simulink model "FMC_TopLevel_Model_2025a"  (R2025a)
settings: Solver=ode23s  StartTime=0.0  StopTime=10.0  RelTol=1e-3
libraries: nesl_utility x1
settings Model: Creator=mu22504  LastModifiedBy=dj23106
settings DataIOCC: InspectSignalLogs=on
settings SimscapeCC: SimscapeLogType=all  SimscapeLogSimulationStatistics=on  SimscapeLogToSDI=on

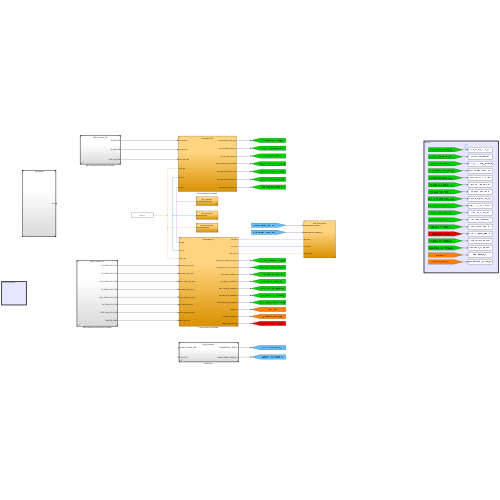
[thumbnail: Simulink's stored preview of the top-level diagram]
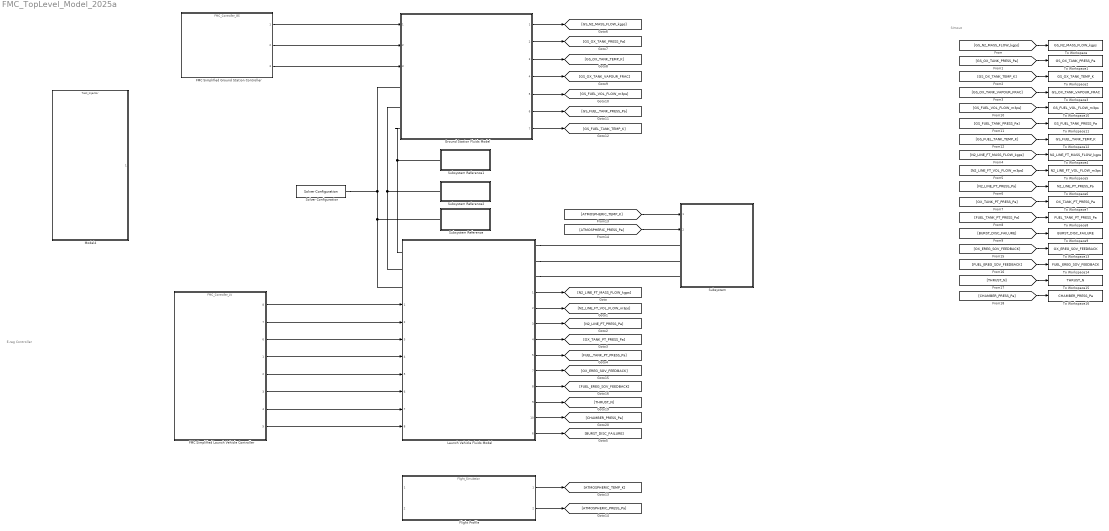
== system FMC_TopLevel_Model_2025a ==
  note: SImout
  note: E-reg Controller
  FMC Simplified Ground Station Controller : ModelReference  ModelNameDialog=FMC_Controller_GS  SimulationMode=Normal  ModelReferenceVersion=1.3
  FMC Simplified Launch Vehicle Controller : ModelReference  ModelNameDialog=FMC_Controller_LV  SimulationMode=Normal  ModelReferenceVersion=1.5
      settings: PortSchema="{\"entries\":[{\"content\":{\"sides\":[{\"content\":{},\"type\":\"ConnectorPlacement.EquallySpacedRectSide\",\"uuid\":\"d1f82117-a1a8-406f-b4c0-5c69a1a9a37f\"},{\"content\":{\"connectorIds\":[\"Out8\",\"Out7\",\"Out6\",\"Out1\",\"Out2\",\"Out3\",\"Out4\",\"Out5\"],\"side\":\"RIGHT\"},\"type\":\"ConnectorPlacement.EquallySpacedRectSide\",\"uuid\":\"19edbef6-afc0-4598-9a4a-36dbc083b03b\"},{\"content\":{\"side\":\"TOP\"},\"type\":\"ConnectorPlacement.EquallySpacedRectSide\",\"uuid\":\"6f6c62f6-4d0e-4b54-92d5-ff51912a203d\"}]},\"type\":\"ConnectorPlacement.EquallySpacedConnector\",\"uuid\":\"dc15e51f-b1bc-449a-a4f6-d80e0204dd3c\"}],\"packageUris\":[\"http://schema.mathworks.com/mf0/Connector/R2020b\"],\"version\":\"1.0\"}"
  "Flight Profile " : ModelReference  ModelNameDialog=Flight_Simulation.slx  SimulationMode=Normal  ModelReferenceVersion=1.3
  Ground Station Fluids Model : Subsystem  ReferencedSubsystem=Thermofluids_GS
      settings: PortSchema="{\"entries\":[{\"content\":{\"sides\":[{\"content\":{\"connectorIds\":[\"In1\",\"In2\",\"In3\",\"LConn3\",\"LConn2\",\"LConn1\"]},\"type\":\"ConnectorPlacement.EquallySpacedRectSide\",\"uuid\":\"1f0e9dc9-066f-4740-a01f-c871041edae1\"},{\"content\":{\"connectorIds\":[\"Out1\",\"Out2\",\"Out3\",\"Out4\",\"Out5\",\"Out6\",\"Out7\"],\"side\":\"RIGHT\"},\"type\":\"ConnectorPlacement.EquallySpacedRectSide\",\"uuid\":\"23696615-9e6b-4b01-bf34-3e6084e0acc4\"},{\"content\":{\"side\":\"TOP\"},\"type\":\"ConnectorPlacement.EquallySpacedRectSide\",\"uuid\":\"47968613-aa29-4234-9156-172438f99733\"}]},\"type\":\"ConnectorPlacement.EquallySpacedConnector\",\"uuid\":\"3d468e28-1aed-4784-9850-3053ce02f939\"}],\"packageUris\":[\"http://schema.mathworks.com/mf0/Connector/R2020b\"],\"version\":\"1.0\"}"
  Launch Vehicle Fluids Model : Subsystem  ReferencedSubsystem=Thermofluids_LV
      settings: PortSchema="{\"entries\":[{\"content\":{\"sides\":[{\"content\":{\"connectorIds\":[\"LConn1\",\"LConn2\",\"LConn3\",\"In1\",\"In2\",\"In3\",\"In4\",\"In5\",\"In6\",\"In7\",\"In8\"]},\"type\":\"ConnectorPlacement.EquallySpacedRectSide\",\"uuid\":\"a87b0425-c6b8-4d08-a1a8-b3acad5c334a\"},{\"content\":{\"connectorIds\":[\"LConn4\",\"LConn5\",\"LConn6\",\"Out1\",\"Out2\",\"Out3\",\"Out4\",\"Out5\",\"Out7\",\"Out8\",\"Out9\",\"Out10\",\"Out6\"],\"side\":\"RIGHT\"},\"type\":\"ConnectorPlacement.EquallySpacedRectSide\",\"uuid\":\"260d6155-6d20-4ed3-9052-698506ea1559\"},{\"content\":{\"side\":\"TOP\"},\"type\":\"ConnectorPlacement.EquallySpacedRectSide\",\"uuid\":\"d266d02d-922b-4f41-b529-513bc445e931\"}]},\"type\":\"ConnectorPlacement.EquallySpacedConnector\",\"uuid\":\"36f51c95-b9e3-4232-bda9-d5a6ea8a2ffc\"}],\"packageUris\":[\"http://schema.mathworks.com/mf0/Connector/R2020b\"],\"version\":\"1.0\"}"
  Model4 : ModelReference  ModelNameDialog=Test_Injector.slx  SimulationMode=Normal  ModelReferenceVersion=1.3
  Solver Configuration : nesl_utility/Solver Configuration  PhysicalDomain=network_engine_domain  SubClassName=solver  LeftPortType=input  RightPortType=generic  Tones=[]  Harmonics=[]  SimulateNoise=off  Profile=off  UseLocalSampling=off  EnableSwitchedLinearOptims=on  FrequencyDomain=off  UseCCode=off  RelTol=0.001  AbsTol=0.001  MinStep=1e-09  ToWorkspace=off  RevertToSquareIcSolve=off  NumHomotopyIterations=100  PhasorMode=off  PhasorModeNumHarmonics=1  ConsistencySolver=NEWTON_XTOL_AFTER_FTOL  IndexReductionMethod=DerivativeReplacement  DoDC=off  ResidualTolerance=1e-09  ConsistencyTolSource=GLOBAL  ConsistencyAbsTol=0.001  ConsistencyRelTol=0.001  ConsistencyTolFactor=0.001  UseLocalSolver=off  LocalSolverChoice=NE_BACKWARD_EULER_ADVANCER  ResolveIndetEquations=on  FunctionEvalNumThread=1  LocalSolverSampleTime=0.001  DoFixedCost=off  MaxNonlinIter=3  MaxModeIter=2  ComputeImpulses=off  ImpulseIterations=2  LinearAlgebra=auto  LinearAlgebraNumThread=0  EquationFormulation=NE_TIME_EF  DelaysMemoryBudget=1024  AutomaticFiltering=on  FilteringTimeConstant=0.001  PartitionStorageMethod=AS_NEEDED  PartitionMemoryBudget=1024  PartitionMethod=ROBUST  MultibodyUseLocalSolver=off  MultibodyLocalSolverChoice=ODE1  MultibodyLocalSolverSampleTime=0.001
  Subsystem : Subsystem  ReferencedSubsystem=Vent_Environment
  Subsystem Reference : Subsystem  ReferencedSubsystem=ethanol_properties
  Subsystem Reference1 : Subsystem  ReferencedSubsystem=N2_properties
  Subsystem Reference2 : Subsystem  ReferencedSubsystem=N2O_properties
  To Workspace : ToWorkspace  VariableName=GS_N2_MASS_FLOW_kgps  SaveFormat=Timeseries  SampleTime=-1
  To Workspace1 : ToWorkspace  VariableName=GS_OX_TANK_PRESS_Pa  SaveFormat=Timeseries  SampleTime=-1
  To Workspace10 : ToWorkspace  VariableName=GS_FUEL_VOL_FLOW_m3ps  SaveFormat=Timeseries  SampleTime=-1
  To Workspace11 : ToWorkspace  VariableName=GS_FUEL_TANK_PRESS_Pa  SaveFormat=Timeseries  SampleTime=-1
  To Workspace12 : ToWorkspace  VariableName=GS_FUEL_TANK_TEMP_K  SaveFormat=Timeseries  SampleTime=-1
  To Workspace13 : ToWorkspace  VariableName=OX_EREG_SOV_FEEDBACK  SaveFormat=Timeseries  SampleTime=-1
  To Workspace14 : ToWorkspace  VariableName=FUEL_EREG_SOV_FEEDBACK  SaveFormat=Timeseries  SampleTime=-1
  To Workspace15 : ToWorkspace  VariableName=THRUST_N  SaveFormat=Timeseries  SampleTime=-1
  To Workspace16 : ToWorkspace  VariableName=CHAMBER_PRESS_Pa  SaveFormat=Timeseries  SampleTime=-1
  To Workspace2 : ToWorkspace  VariableName=GS_OX_TANK_TEMP_K  SaveFormat=Timeseries  SampleTime=-1
  To Workspace3 : ToWorkspace  VariableName=GS_OX_TANK_VAPOUR_FRAC  SaveFormat=Timeseries  SampleTime=-1
  To Workspace4 : ToWorkspace  VariableName=N2_LINE_FT_MASS_FLOW_kgps  SaveFormat=Timeseries  SampleTime=-1
  To Workspace5 : ToWorkspace  VariableName=N2_LINE_FT_VOL_FLOW_m3ps  SaveFormat=Timeseries  SampleTime=-1
  To Workspace6 : ToWorkspace  VariableName=N2_LINE_PT_PRESS_Pa  SaveFormat=Timeseries  SampleTime=-1
  To Workspace7 : ToWorkspace  VariableName=OX_TANK_PT_PRESS_Pa  SaveFormat=Timeseries  SampleTime=-1
  To Workspace8 : ToWorkspace  VariableName=FUEL_TANK_PT_PRESS_Pa  SaveFormat=Timeseries  SampleTime=-1
  To Workspace9 : ToWorkspace  VariableName=BURST_DISC_FAILURE  SaveFormat=Timeseries  SampleTime=-1
  wires:
  Launch Vehicle Fluids Model/1 -> [N2_LINE_FT_MASS_FLOW_kgps]
  Launch Vehicle Fluids Model/2 -> [N2_LINE_FT_VOL_FLOW_m3ps]
  Launch Vehicle Fluids Model/3 -> [N2_LINE_PT_PRESS_Pa]
  Launch Vehicle Fluids Model/4 -> [OX_TANK_PT_PRESS_Pa]
  Launch Vehicle Fluids Model/5 -> [FUEL_TANK_PT_PRESS_Pa]
  Launch Vehicle Fluids Model/6 -> [BURST_DISC_FAILURE]
  FMC Simplified Ground Station Controller/1 -> Ground Station Fluids Model/1
  FMC Simplified Ground Station Controller/2 -> Ground Station Fluids Model/2
  FMC Simplified Ground Station Controller/3 -> Ground Station Fluids Model/3
  Ground Station Fluids Model/1 -> [GS_N2_MASS_FLOW_kgps]
  Ground Station Fluids Model/2 -> [GS_OX_TANK_PRESS_Pa]
  Ground Station Fluids Model/3 -> [GS_OX_TANK_TEMP_K]
  Ground Station Fluids Model/4 -> [GS_OX_TANK_VAPOUR_FRAC]
  [GS_N2_MASS_FLOW_kgps] -> To Workspace/1
  [GS_OX_TANK_PRESS_Pa] -> To Workspace1/1
  [GS_OX_TANK_TEMP_K] -> To Workspace2/1
  [GS_OX_TANK_VAPOUR_FRAC] -> To Workspace3/1
  [N2_LINE_FT_MASS_FLOW_kgps] -> To Workspace4/1
  [BURST_DISC_FAILURE] -> To Workspace9/1
  [FUEL_TANK_PT_PRESS_Pa] -> To Workspace8/1
  [OX_TANK_PT_PRESS_Pa] -> To Workspace7/1
  [N2_LINE_PT_PRESS_Pa] -> To Workspace6/1
  [N2_LINE_FT_VOL_FLOW_m3ps] -> To Workspace5/1
  FMC Simplified Launch Vehicle Controller/5 -> Launch Vehicle Fluids Model/8
  FMC Simplified Launch Vehicle Controller/4 -> Launch Vehicle Fluids Model/7
  FMC Simplified Launch Vehicle Controller/3 -> Launch Vehicle Fluids Model/6
  FMC Simplified Launch Vehicle Controller/2 -> Launch Vehicle Fluids Model/5
  FMC Simplified Launch Vehicle Controller/1 -> Launch Vehicle Fluids Model/4
  FMC Simplified Launch Vehicle Controller/6 -> Launch Vehicle Fluids Model/3
  FMC Simplified Launch Vehicle Controller/7 -> Launch Vehicle Fluids Model/2
  FMC Simplified Launch Vehicle Controller/8 -> Launch Vehicle Fluids Model/1
  Ground Station Fluids Model/5 -> [GS_FUEL_VOL_FLOW_m3ps]
  Ground Station Fluids Model/6 -> [GS_FUEL_TANK_PRESS_Pa]
  Ground Station Fluids Model/7 -> [GS_FUEL_TANK_TEMP_K]
  [GS_FUEL_VOL_FLOW_m3ps] -> To Workspace10/1
  [GS_FUEL_TANK_PRESS_Pa] -> To Workspace11/1
  [GS_FUEL_TANK_TEMP_K] -> To Workspace12/1
  "Flight Profile "/1 -> [ATMOSPHERIC_TEMP_K]
  "Flight Profile "/2 -> [ATMOSPHERIC_PRESS_Pa]
  [ATMOSPHERIC_TEMP_K] -> Subsystem/1
  [ATMOSPHERIC_PRESS_Pa] -> Subsystem/2
  Launch Vehicle Fluids Model/7 -> [OX_EREG_SOV_FEEDBACK]
  Launch Vehicle Fluids Model/8 -> [FUEL_EREG_SOV_FEEDBACK]
  [OX_EREG_SOV_FEEDBACK] -> To Workspace13/1
  [FUEL_EREG_SOV_FEEDBACK] -> To Workspace14/1
  Launch Vehicle Fluids Model/9 -> [THRUST_N]
  Launch Vehicle Fluids Model/10 -> [CHAMBER_PRESS_Pa]
  [THRUST_N] -> To Workspace15/1
  [CHAMBER_PRESS_Pa] -> To Workspace16/1
  connections:
  Ground Station Fluids Model/LConn1 -- Subsystem Reference1/LConn1 -- Launch Vehicle Fluids Model/LConn1
  Launch Vehicle Fluids Model/LConn2 -- Subsystem Reference2/LConn1 -- Ground Station Fluids Model/LConn2
  Launch Vehicle Fluids Model/LConn3 -- Subsystem Reference/LConn1 -- Solver Configuration/RConn1 -- Ground Station Fluids Model/LConn3
  Launch Vehicle Fluids Model/LConn4 -- Subsystem/LConn1
  Launch Vehicle Fluids Model/LConn5 -- Subsystem/LConn2
  Launch Vehicle Fluids Model/LConn6 -- Subsystem/LConn3
